simulink model "EV_range_estimation"  (R2022b)
settings: Solver=ode45  StartTime=0.0  StopTime=1874  MaxStep=1e-2  RelTol=1e-3
settings Model: Creator=adity  LastModifiedBy=adity

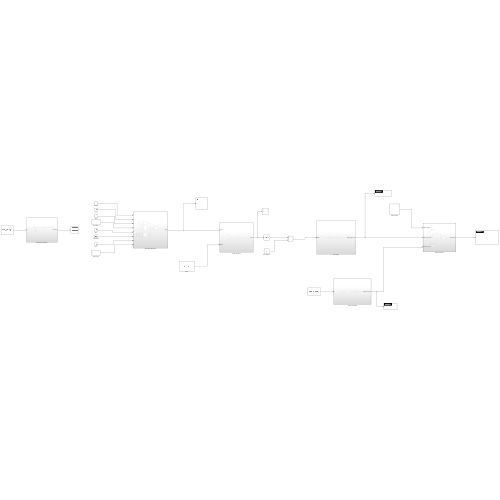
[thumbnail: Simulink's stored preview of the top-level diagram]
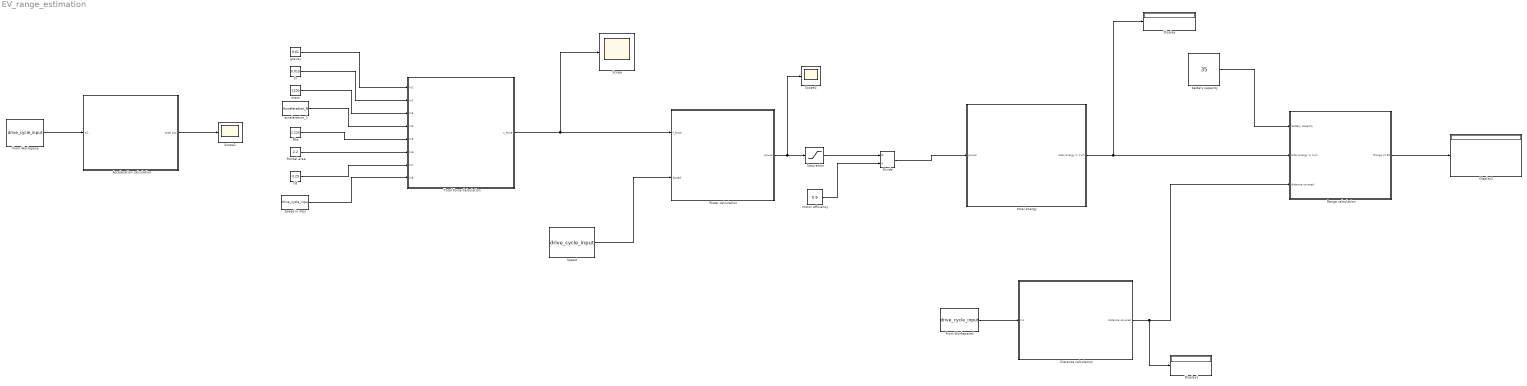
== system EV_range_estimation ==
  Acceleration calculation : Subsystem
  Cd : Constant  Value=0.29
  Cr : Constant  Value=0.015
  Display : Display
  Display1 : Display
  Display2 : Display
  Distance calculation : Subsystem
  Divide : Product  Inputs=*/
  From Workspace : FromWorkspace  VariableName=drive_cycle_input  SampleTime=1
  From Workspace1 : FromWorkspace  VariableName=drive_cycle_input  SampleTime=1
  Power calculation : Subsystem
  Range calculation : Subsystem
  Rho : Constant  Value=1.225
  Saturation : Saturate  UpperLimit=Inf  LowerLimit=0
  Scope : Scope
  Scope1 : Scope
  Scope2 : Scope
  Speed : FromWorkspace  VariableName=drive_cycle_input  SampleTime=1
  Total Force Calculation : Subsystem
  acceleration_1 : FromWorkspace  VariableName=Acceleration_N  SampleTime=1
  battery capacity : Constant  Value=35
  frontal area : Constant  Value=2.2
  gravity : Constant  Value=9.81
  mass : Constant  Value=1200
  motor efficiency : Constant  Value=0.9
  speed in mps : FromWorkspace  VariableName=drive_cycle_input  SampleTime=1
  total energy : Subsystem
  wires:
  gravity/1 -> Total Force Calculation/1(In1)
  Cr/1 -> Total Force Calculation/2(In2)
  mass/1 -> Total Force Calculation/3(In3)
  acceleration_1/1 -> Total Force Calculation/4(In4)
  Rho/1 -> Total Force Calculation/5(In5)
  frontal area/1 -> Total Force Calculation/6(In6)
  Cd/1 -> Total Force Calculation/7(In7)
  speed in mps/1 -> Total Force Calculation/8(In8)
  Speed/1 -> Power calculation/2(Speed)
  Total Force Calculation/1(t_force) -> Scope/1, Power calculation/1(t_force)
  From Workspace1/1 -> Distance calculation/1(In1)
  battery capacity/1 -> Range calculation/1(battery capacity)
  total energy/1(total energy in kwh) -> Display/1, Range calculation/2(total energy in kwh)
  Distance calculation/1(distance covered) -> Display1/1, Range calculation/3(distance covered)
  Range calculation/1(Range of EV) -> Display2/1
  Power calculation/1(power) -> Scope2/1, Saturation/1
  Saturation/1 -> Divide/1
  motor efficiency/1 -> Divide/2
  Divide/1 -> total energy/1(power)
  From Workspace/1 -> Acceleration calculation/1(In1)
  Acceleration calculation/1(total acc) -> Scope1/1

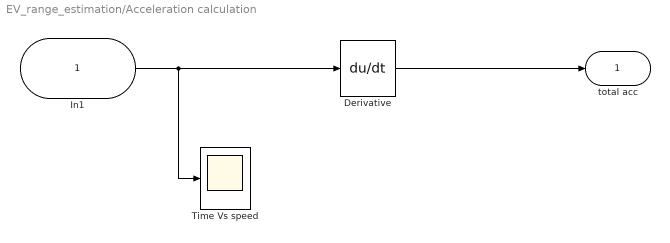
== system EV_range_estimation/Acceleration calculation ==
  In1 : Inport
  Derivative : Derivative
  Time Vs speed : Scope
  total acc : Outport
  wires:
  In1/1 -> Time Vs speed/1, Derivative/1
  Derivative/1 -> total acc/1

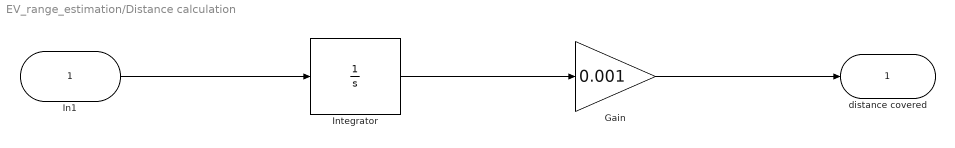
== system EV_range_estimation/Distance calculation ==
  In1 : Inport
  Gain : Gain  Gain=0.001
  Integrator : Integrator
  distance covered : Outport
  wires:
  In1/1 -> Integrator/1
  Integrator/1 -> Gain/1
  Gain/1 -> distance covered/1

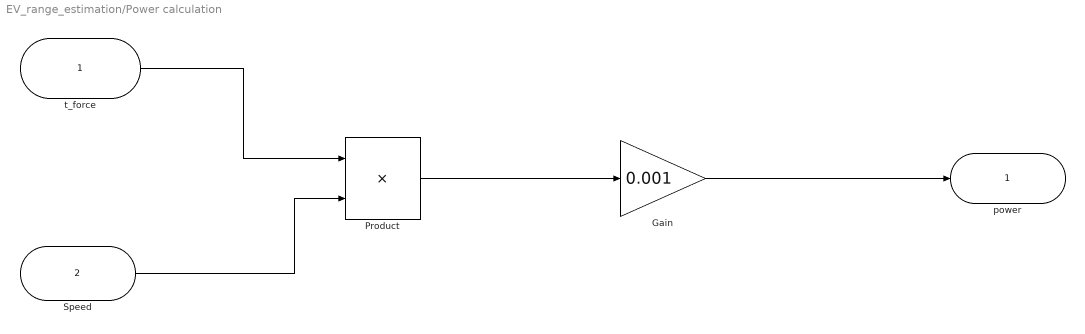
== system EV_range_estimation/Power calculation ==
  t_force : Inport
  Speed : Inport  Port=2
  Gain : Gain  Gain=0.001
  Product : Product
  power : Outport
  wires:
  t_force/1 -> Product/1
  Speed/1 -> Product/2
  Product/1 -> Gain/1
  Gain/1 -> power/1

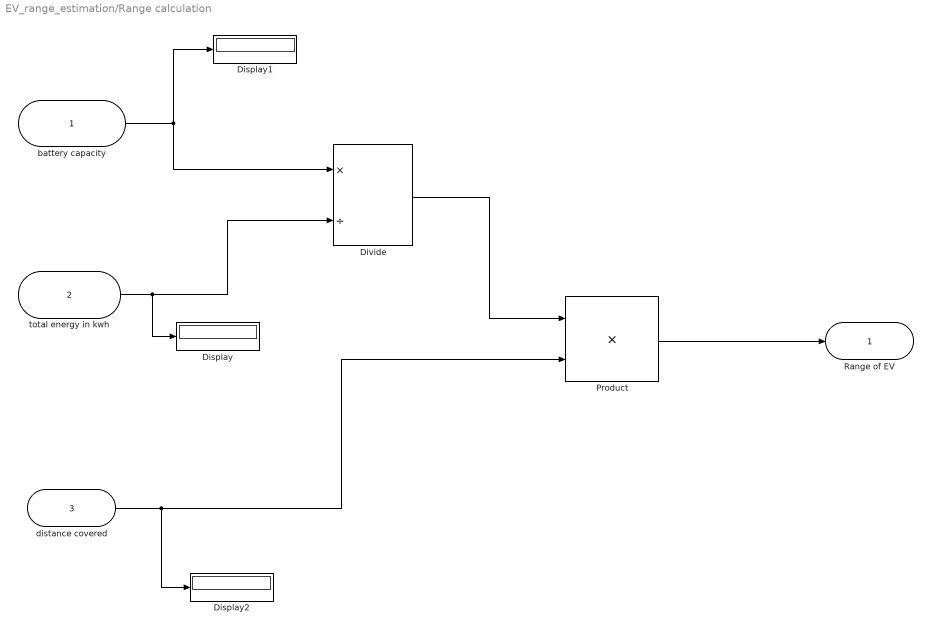
== system EV_range_estimation/Range calculation ==
  battery capacity : Inport
  total energy in kwh : Inport  Port=2
  distance covered : Inport  Port=3
  Display : Display
  Display1 : Display
  Display2 : Display
  Divide : Product  Inputs=*/
  Product : Product
  Range of EV : Outport
  wires:
  battery capacity/1 -> Display1/1, Divide/1
  distance covered/1 -> Display2/1, Product/2
  Product/1 -> Range of EV/1
  Divide/1 -> Product/1
  total energy in kwh/1 -> Display/1, Divide/2

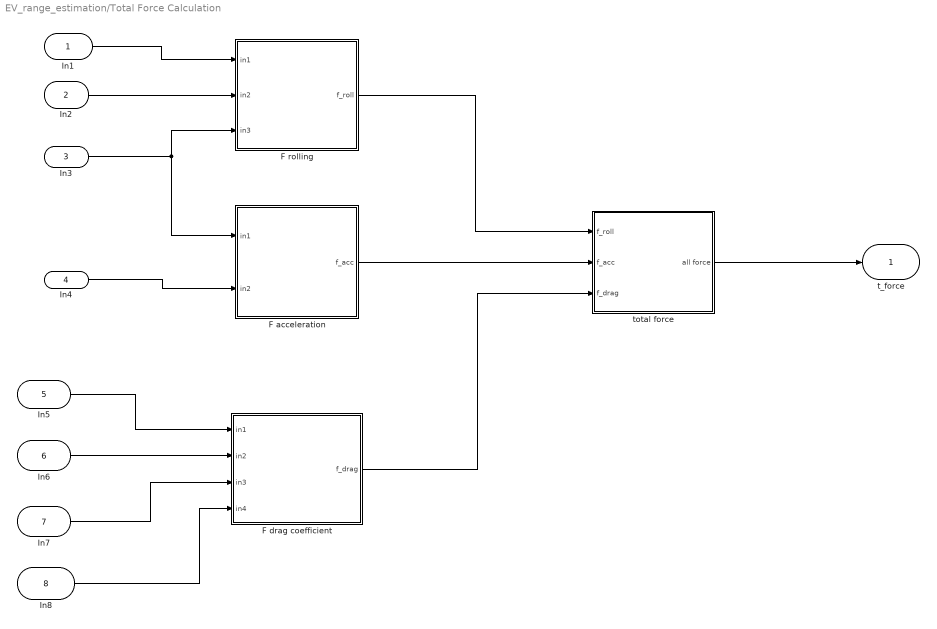
== system EV_range_estimation/Total Force Calculation ==
  In1 : Inport
  In2 : Inport  Port=2
  In3 : Inport  Port=3
  In4 : Inport  Port=4
  In5 : Inport  Port=5
  In6 : Inport  Port=6
  In7 : Inport  Port=7
  In8 : Inport  Port=8
  F acceleration : Subsystem
  F drag coefficient : Subsystem
  F rolling : Subsystem
  total force : Subsystem
  t_force : Outport
  wires:
  total force/1(all force) -> t_force/1
  In1/1 -> F rolling/1(in1)
  In2/1 -> F rolling/2(in2)
  In3/1 -> F acceleration/1(in1), F rolling/3(in3)
  In4/1 -> F acceleration/2(in2)
  In5/1 -> F drag coefficient/1(in1)
  In6/1 -> F drag coefficient/2(in2)
  In7/1 -> F drag coefficient/3(in3)
  In8/1 -> F drag coefficient/4(in4)
  F rolling/1(f_roll) -> total force/1(f_roll)
  F acceleration/1(f_acc) -> total force/2(f_acc)
  F drag coefficient/1(f_drag) -> total force/3(f_drag)

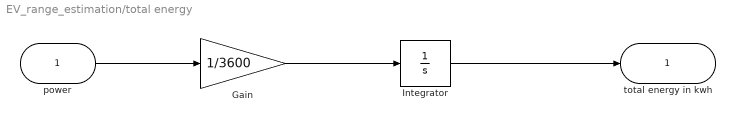
== system EV_range_estimation/total energy ==
  power : Inport
  Gain : Gain  Gain=1/3600
  Integrator : Integrator
  total energy in kwh : Outport
  wires:
  power/1 -> Gain/1
  Gain/1 -> Integrator/1
  Integrator/1 -> total energy in kwh/1

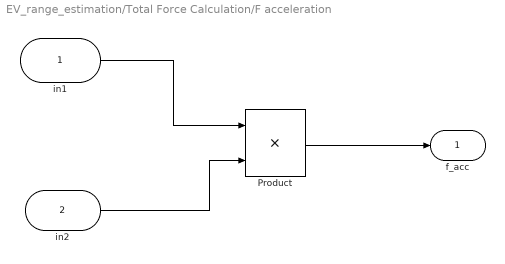
== system EV_range_estimation/Total Force Calculation/F acceleration ==
  in1 : Inport
  in2 : Inport  Port=2
  Product : Product
  f_acc : Outport
  wires:
  in1/1 -> Product/1
  in2/1 -> Product/2
  Product/1 -> f_acc/1

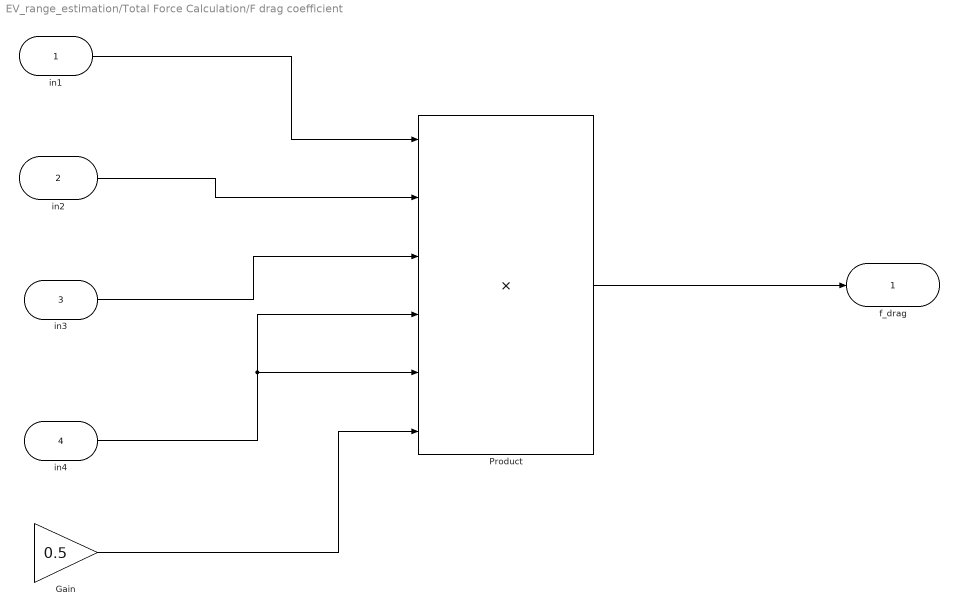
== system EV_range_estimation/Total Force Calculation/F drag coefficient ==
  in1 : Inport
  in2 : Inport  Port=2
  in3 : Inport  Port=3
  in4 : Inport  Port=4
  Gain : Gain  Gain=0.5
  Product : Product  Inputs=6
  f_drag : Outport
  wires:
  in1/1 -> Product/1
  in2/1 -> Product/2
  in3/1 -> Product/3
  in4/1 -> Product/5, Product/4
  Gain/1 -> Product/6
  Product/1 -> f_drag/1

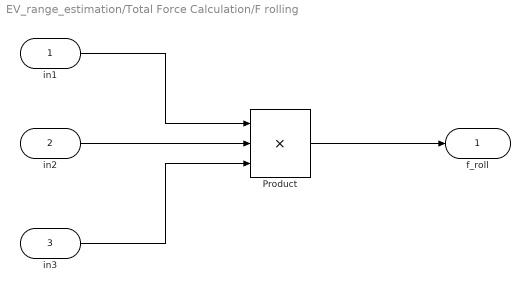
== system EV_range_estimation/Total Force Calculation/F rolling ==
  in1 : Inport
  in2 : Inport  Port=2
  in3 : Inport  Port=3
  Product : Product  Inputs=3
  f_roll : Outport
  wires:
  in1/1 -> Product/1
  in2/1 -> Product/2
  in3/1 -> Product/3
  Product/1 -> f_roll/1

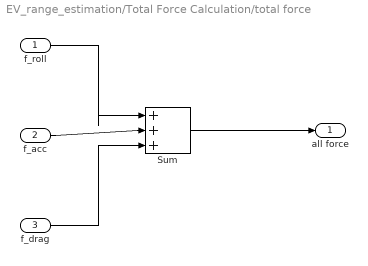
== system EV_range_estimation/Total Force Calculation/total force ==
  f_roll : Inport
  f_acc : Inport  Port=2
  f_drag : Inport  Port=3
  Sum : Sum  Inputs=|+++
  all force : Outport
  wires:
  f_roll/1 -> Sum/1
  f_acc/1 -> Sum/2
  f_drag/1 -> Sum/3
  Sum/1 -> all force/1
